simulink model "modelWachadla_v2"  (R2017a)
settings: Solver=VariableStepAuto  StartTime=0.0  StopTime=100  MinStep=0.01  RelTol=1e-3  EnableMultiTasking=on
undefined symbols (not defined in the file or in its folder): A0, A135, A180, A45, A90, B0, B135, B180, B45, B90
libraries: fuzblock x1
settings Model: Creator=student  LastModifiedBy=Szwank
settings DataIOCC: SaveFormat=StructureWithTime
settings OptimizationCC: LifeSpan=inf
settings DebuggingCC: SFUnexpectedBacktrackingDiag=warning  SFNoUnconditionalDefaultTransitionDiag=warning  SFExecutionAtInitializationDiag=none
settings HardwareCC: ProdBitPerSizeT=32  ProdBitPerPtrDiffT=32  ProdWordSize=32  ProdHWDeviceType=Specified
settings GRTTargetCC: TargetLangStandard=C89/C90 (ANSI)  GeneratePreprocessorConditionals=Disable all
settings ConfigComp: CovMetricSettings=dw  CovHtmlReporting=on  CovSaveCumulativeToWorkspaceVar=on  CovSaveSingleToWorkspaceVar=on  CovExternalEMLEnable=off

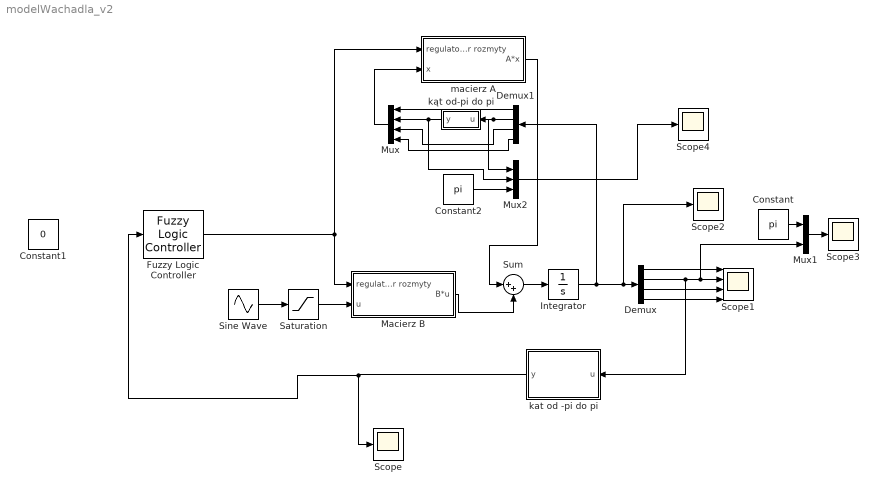
== system modelWachadla_v2 ==
  Constant : Constant  Value=pi
  Constant1 : Constant  Value=0
  Constant2 : Constant  Value=pi
  Demux : Demux
  Demux1 : Demux
  Fuzzy Logic Controller : fuzblock/Fuzzy Logic  Controller  fis=['modelRozmyty_v2.fis']
  Integrator : Integrator  InitialCondition=[0 pi 0 0]
  Macierz B : Subsystem
  Mux : Mux
  Mux1 : Mux  Inputs=2
  Mux2 : Mux  Inputs=3
  Saturation : Saturate  UpperLimit=10  LowerLimit=-10
  Scope{,2..4} (4 alike) : Scope
  Scope1 : Scope  NumInputPorts=4
  Sine Wave : Sin  Amplitude=0.1  Frequency=0.1  SampleTime=0
  Sum : Sum  Inputs=|++
  kat od -pi do pi : MATLAB Function  TreatAsAtomicUnit=on
  kąt od-pi do pi : MATLAB Function  TreatAsAtomicUnit=on
  "macierz A " : Subsystem
  wires:
  Sum/1 -> Integrator/1
  Demux/2 -> kat od -pi do pi/1(u), Mux1/2, Scope1/2
  "macierz A "/1(A*x) -> Sum/1
  Macierz B/1(B*u) -> Sum/2
  Demux/1 -> Scope1/1
  Demux/3 -> Scope1/3
  Demux/4 -> Scope1/4
  kat od -pi do pi/1(y) -> Fuzzy Logic Controller/1, Scope/1
  Fuzzy Logic Controller/1 -> Macierz B/1("regulator rozmyty "), "macierz A "/1(regulator rozmyty)
  Integrator/1 -> Scope2/1, Demux/1, Demux1/1
  Demux1/4 -> Mux/4
  Demux1/2 -> kąt od-pi do pi/1(u), Mux2/1
  Demux1/3 -> Mux/3
  Demux1/1 -> Mux/1
  Mux/1 -> "macierz A "/2("x ")
  Mux1/1 -> Scope3/1
  Constant/1 -> Mux1/1
  Mux2/1 -> Scope4/1
  Constant2/1 -> Mux2/3
  Saturation/1 -> Macierz B/2("u ")
  kąt od-pi do pi/1(y) -> Mux2/2, Mux/2
  Sine Wave/1 -> Saturation/1

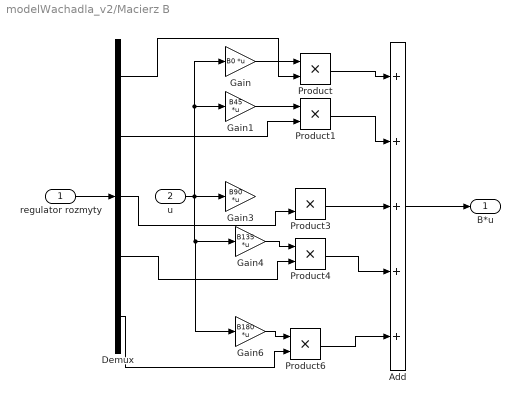
== system modelWachadla_v2/Macierz B ==
  "regulator rozmyty " : Inport
  "u " : Inport  Port=2
  Add : Sum  Inputs=+++++
  Demux : Demux  Outputs=5
  Gain : Gain  Gain=B0  Multiplication=Matrix(K*u)
  Gain1 : Gain  Gain=B45  Multiplication=Matrix(K*u)
  Gain3 : Gain  Gain=B90  Multiplication=Matrix(K*u)
  Gain4 : Gain  Gain=B135  Multiplication=Matrix(K*u)
  Gain6 : Gain  Gain=B180  Multiplication=Matrix(K*u)
  Product{,1,3..4,6} (5 alike) : Product
  B*u : Outport
  wires:
  "regulator rozmyty "/1 -> Demux/1
  Add/1 -> B*u/1
  Demux/1 -> Product/2
  "u "/1 -> Gain6/1, Gain4/1, Gain1/1, Gain/1, Gain3/1
  Demux/2 -> Product1/2
  Product/1 -> Add/1
  Product1/1 -> Add/2
  Gain6/1 -> Product6/1
  Demux/3 -> Product3/2
  Demux/4 -> Product4/2
  Demux/5 -> Product6/2
  Product3/1 -> Add/3
  Product4/1 -> Add/4
  Product6/1 -> Add/5
  Gain4/1 -> Product4/1
  Gain1/1 -> Product1/1
  Gain/1 -> Product/1

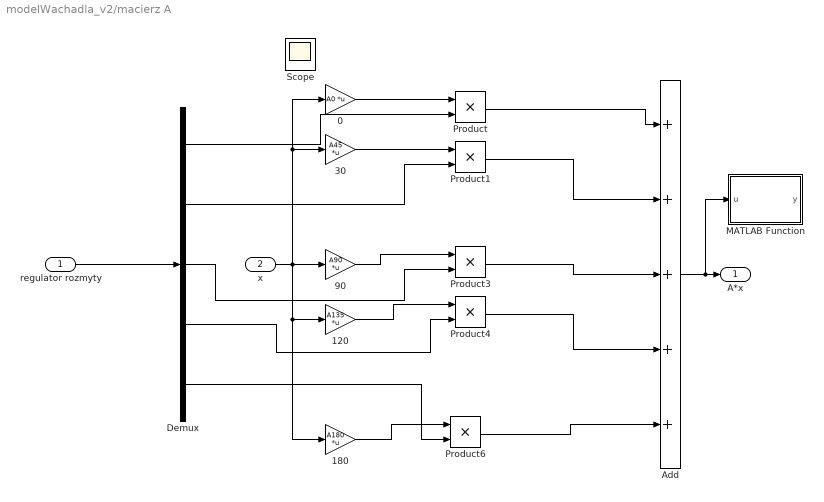
== system modelWachadla_v2/macierz A  ==
  regulator rozmyty : Inport
  "x " : Inport  Port=2
  0 : Gain  Gain=A0  Multiplication=Matrix(K*u)
  120 : Gain  Gain=A135  Multiplication=Matrix(K*u)
  180 : Gain  Gain=A180  Multiplication=Matrix(K*u)
  "30 " : Gain  Gain=A45  Multiplication=Matrix(K*u)
  90 : Gain  Gain=A90  Multiplication=Matrix(K*u)
  Add : Sum  Inputs=+++++
  Demux : Demux  Outputs=5
  MATLAB Function : MATLAB Function  TreatAsAtomicUnit=on
  Product{,1,3..4,6} (5 alike) : Product
  Scope : Scope
  A*x : Outport
  wires:
  regulator rozmyty/1 -> Demux/1
  Add/1 -> MATLAB Function/1(u), A*x/1
  "x "/1 -> 120/1, 180/1, 0/1, "30 "/1, 90/1
  Product/1 -> Add/1
  Product1/1 -> Add/2
  180/1 -> Product6/1
  Demux/1 -> Product/2
  Demux/2 -> Product1/2
  Demux/3 -> Product3/2
  Demux/4 -> Product4/2
  Demux/5 -> Product6/2
  Product3/1 -> Add/3
  Product4/1 -> Add/4
  Product6/1 -> Add/5
  120/1 -> Product4/1
  90/1 -> Product3/1
  "30 "/1 -> Product1/1
  0/1 -> Product/1

== matlab function modelWachadla_v2/kąt od-pi do pi ==
  data: u input; y output
function y = fcn(u)

u=rem(u,2*pi);


if(u>0)
    u=rem(u,2*pi);
    if(u>pi)
        u=-pi+rem(u,pi);
    end
end

if(u<0)
    u=rem(u,2*pi);
    if(u<-pi)
        u=pi+rem(u,pi);
    end
end
y = u;

== matlab function modelWachadla_v2/macierz A /MATLAB Function ==
  data: u input; y output
function y = fcn(u)

y = u;

== matlab function modelWachadla_v2/kat od -pi do pi ==
  data: u input; y output
function y = fcn(u)

u=rem(u,2*pi);


if(u>0)
    if(u>pi)
        u=-pi+rem(u,pi);
    end
end

if(u<0)
    if(u<-pi)
        u=pi+rem(u,pi);
    end
end
y = u;
